simulink model "testsim"  (R2019a)
settings: Solver=ode45  StartTime=0.0  StopTime=3.0  RelTol=1e-3
values from neighbouring files (symbols this model uses):
  currentX = Swarm.Particles(k).X    [test.m]
settings Model: Creator=Sombit Roy  LastModifiedBy=Sombit Roy
settings SolverCC: MaxConsecutiveMinStep=2
settings DataIOCC: ReturnWorkspaceOutputs=off

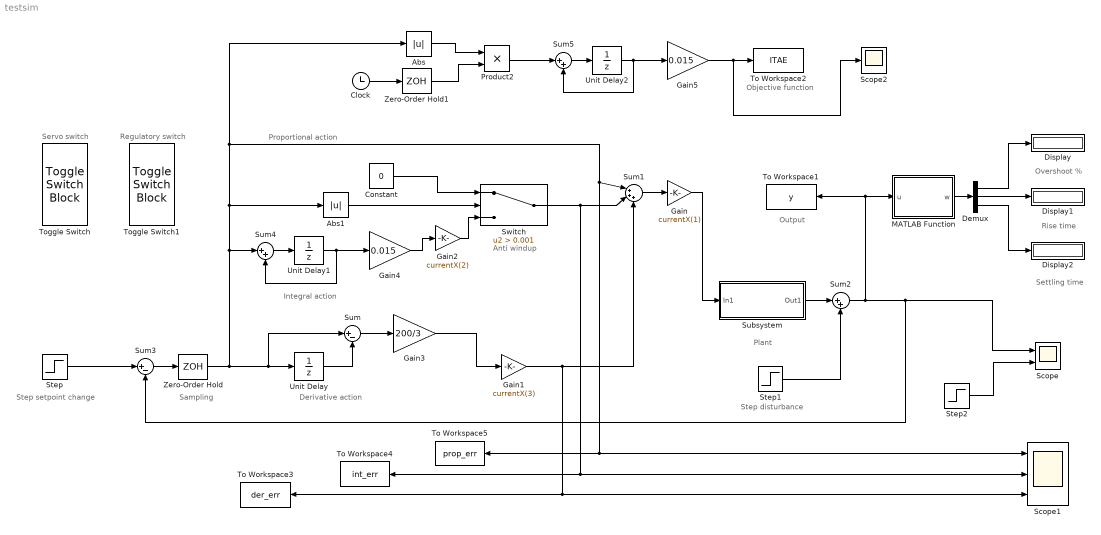
== system testsim ==
  note: Settling time
  note: Rise time
  note: Overshoot %
  note: Output
  note: Sampling
  note: Step setpoint change
  note: Step disturbance
  note: Plant
  note: Anti windup
  note: Objective function
  note: Proportional action
  note: Integral action
  note: Derivative action
  note: Regulatory switch
  note: Servo switch
  Abs : Abs
  Abs1 : Abs
  Clock : Clock
  Constant : Constant  Value=0
  Demux : Demux  Outputs=3
  Display : Display
  Display1 : Display
  Display2 : Display
  Gain : Gain  Gain=currentX(1)
  Gain1 : Gain  Gain=currentX(3)
  Gain2 : Gain  Gain=currentX(2)
  Gain3 : Gain  Gain=200/3
  Gain4 : Gain  Gain=0.015
  Gain5 : Gain  Gain=0.015
  MATLAB Function : MATLAB Function  TreatAsAtomicUnit=on
  Product2 : Product
  Scope : Scope  NumInputPorts=2
  Scope1 : Scope  NumInputPorts=3
  Scope2 : Scope
  Step : Step  SampleTime=0
  Step1 : Step  After=0  SampleTime=0
  Step2 : Step  SampleTime=0
  Subsystem : Subsystem
  Sum : Sum  Inputs=|+-
  Sum1 : Sum  Inputs=|+++
  Sum2 : Sum  Inputs=|++
  Sum3 : Sum  Inputs=|+-
  Sum4 : Sum  Inputs=|++
  Sum5 : Sum  Inputs=|++
  Switch : Switch  Criteria=u2 > Threshold  Threshold=0.001
  To Workspace1 : ToWorkspace  VariableName=y  SaveFormat=Timeseries  SampleTime=-1
  To Workspace2 : ToWorkspace  VariableName=ITAE  SaveFormat=Timeseries  SampleTime=-1
  To Workspace3 : ToWorkspace  VariableName=der_err  SaveFormat=Timeseries  SampleTime=-1
  To Workspace4 : ToWorkspace  VariableName=int_err  SaveFormat=Timeseries  SampleTime=-1
  To Workspace5 : ToWorkspace  VariableName=prop_err  SaveFormat=Timeseries  SampleTime=-1
  Toggle Switch : ToggleSwitchBlock  LabelPosition=Hide
      settings: Values={{'Off', 'On'}, [0 1]}
  Toggle Switch1 : ToggleSwitchBlock  LabelPosition=Hide
      settings: Values={{'Off', 'On'}, [0 1]}
  Unit Delay : UnitDelay  SampleTime=0.015  HasFrameUpgradeWarning=on
  Unit Delay1 : UnitDelay  SampleTime=0.015  HasFrameUpgradeWarning=on
  Unit Delay2 : UnitDelay  SampleTime=0.015  HasFrameUpgradeWarning=on
  Zero-Order Hold : ZeroOrderHold  SampleTime=0.015
  Zero-Order Hold1 : ZeroOrderHold  SampleTime=0.015
  wires:
  Zero-Order Hold/1 -> Sum/1, Unit Delay/1, Sum1/1, To Workspace5/1, Scope1/1, Abs/1, Abs1/1, Sum4/1
  Step/1 -> Sum3/1
  Abs/1 -> Product2/1
  Gain5/1 -> Scope2/1, To Workspace2/1
  Switch/1 -> Sum1/2, To Workspace4/1, Scope1/2
  Gain/1 -> Subsystem/1(In1)
  Sum1/1 -> Gain/1
  Gain1/1 -> Sum1/3, To Workspace3/1, Scope1/3
  Gain2/1 -> Switch/3
  Constant/1 -> Switch/1
  Subsystem/1(Out1) -> Sum2/1
  Sum2/1 -> Sum3/2, Scope/1, MATLAB Function/1(u), To Workspace1/1
  Step1/1 -> Sum2/2
  Step2/1 -> Scope/2
  Sum3/1 -> Zero-Order Hold/1
  Unit Delay/1 -> Sum/2
  Sum/1 -> Gain3/1
  Gain3/1 -> Gain1/1
  Sum4/1 -> Unit Delay1/1
  Unit Delay1/1 -> Gain4/1, Sum4/2
  Gain4/1 -> Gain2/1
  Zero-Order Hold1/1 -> Product2/2
  Clock/1 -> Zero-Order Hold1/1
  Product2/1 -> Sum5/1
  Sum5/1 -> Unit Delay2/1
  Unit Delay2/1 -> Gain5/1, Sum5/2
  Abs1/1 -> Switch/2
  MATLAB Function/1(w) -> Demux/1
  Demux/1 -> Display/1
  Demux/2 -> Display1/1
  Demux/3 -> Display2/1

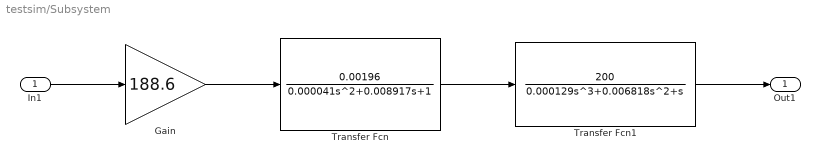
== system testsim/Subsystem ==
  In1 : Inport
  Gain : Gain  Gain=188.6
  Transfer Fcn : TransferFcn  Numerator=[0.00196]  Denominator=[0.000041 0.008917 1]
  Transfer Fcn1 : TransferFcn  Numerator=[200]  Denominator=[0.000129 0.006818 1 0]
  Out1 : Outport
  wires:
  Transfer Fcn/1 -> Transfer Fcn1/1
  Transfer Fcn1/1 -> Out1/1
  Gain/1 -> Transfer Fcn/1
  In1/1 -> Gain/1

== matlab function testsim/MATLAB Function ==
  settings: updateMethod=DISCRETE
  data: u input; w output
function w = performance(u)

    persistent n
    if isempty(n)
        n = 0;
    end
    n = n+1;

    persistent overshoot
    if isempty(overshoot)
        overshoot = 0;
    end
    if (u-1)*100 > overshoot
        overshoot = (u-1)*100;
    end

    persistent flag
    if isempty(flag)
        flag = 0;
    end

    persistent rise
    if isempty(rise)
        rise = 0;
    end
    if flag == 0 && u > 1
        rise = n/201*3 - 1;
        flag = 1;
    end

    persistent settling
    if isempty(settling)
        settling = 0;
    end

    if (u > 1.002 || u < 0.998)
        settling = n/201*3 - 1;
    end

    w = [overshoot rise settling];

end
